simulink model "ipmsm_mechanical_test"  (R2015a)
settings: Solver=ode45  StartTime=0.0  StopTime=0.05  RelTol=1e-3
settings Model: Creator=user  LastModifiedBy=user

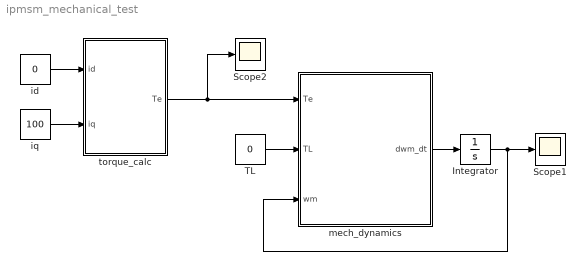
== system ipmsm_mechanical_test ==
  Integrator : Integrator
  Scope1 : Scope
  Scope2 : Scope
  TL : Constant  Value=0
  id : Constant  Value=0
  iq : Constant  Value=100
  mech_dynamics : MATLAB Function  TreatAsAtomicUnit=on
  torque_calc : MATLAB Function  TreatAsAtomicUnit=on
  wires:
  id/1 -> torque_calc/1(id)
  iq/1 -> torque_calc/2(iq)
  torque_calc/1(Te) -> Scope2/1, mech_dynamics/1(Te)
  TL/1 -> mech_dynamics/2(TL)
  mech_dynamics/1(dwm_dt) -> Integrator/1
  Integrator/1 -> Scope1/1, mech_dynamics/3(wm)

== matlab function ipmsm_mechanical_test/mech_dynamics ==
  data: Te input; dwm_dt output; TL input; wm input
function dwm_dt = mech_dynamics(Te, TL, wm)
% BMW i3 mechanical dynamics
% Units: Te, TL in Nm; wm in rad/s; dwm_dt in rad/s^2

J = 0.06;    % ASSUMED
B = 0.001;   % ASSUMED

dwm_dt = (Te - TL - B*wm) / J;

end

== matlab function ipmsm_mechanical_test/torque_calc ==
  data: id input; Te output; iq input
function Te = torque_calc(id, iq)
% BMW i3 electromagnetic torque
% Units: id, iq in A; Te in Nm

Ld       = 0.090e-3;
Lq       = 0.255e-3;
lambda_m = 0.0385;
p        = 6;

Te = (3/2) * p * (lambda_m*iq + (Ld - Lq)*id*iq);

end
